simulink model "shabih_model"  (R2021a)
settings: Solver=VariableStepAuto  StartTime=0.0  StopTime=20  MaxStep=0.1  RelTol=1e-3
libraries: cstblocks x3, pid_lib x1
settings Model: Creator=saeed  LastModifiedBy=saeed

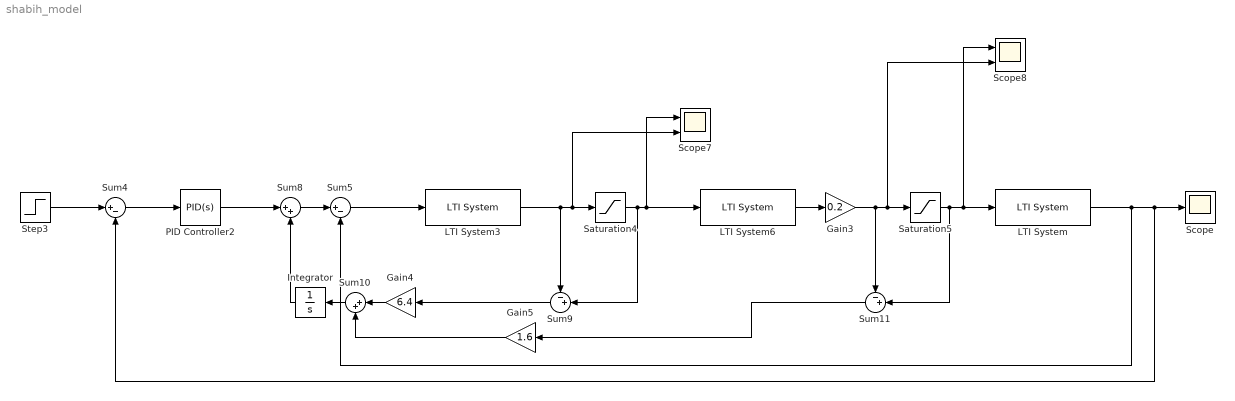
== system shabih_model ==
  Gain3 : Gain  Gain=0.2
  Gain4 : Gain  Gain=6.4
  Gain5 : Gain  Gain=1.6
  Integrator : Integrator
  LTI System : cstblocks/LTI System  sys=G_plant  IC=[]
  LTI System3 : cstblocks/LTI System  sys=C  IC=[]
  LTI System6 : cstblocks/LTI System  sys=G_motor  IC=[]
  PID Controller2 : pid_lib/PID Controller  Controller=PID  Form=Parallel  TimeDomain=Continuous-time  UseExternalTs=off  SampleTime=-1  IntegratorMethod=Forward Euler  FilterMethod=Forward Euler  ControllerParametersSource=internal  P=0.191923492855687  I=0.488933359561099  D=0  UseFilter=on  N=100  TunerSelectOption=Transfer Function Based (PID Tuner App)  InitialConditionSource=internal  InitialConditionForIntegrator=0  InitialConditionForFilter=0  DifferentiatorICPrevScaledInput=0  ExternalReset=none  TrackingMode=off  Kt=1  LimitOutput=on  SatLimitsSource=internal  UpperSaturationLimit=inf  LowerSaturationLimit=-inf  LinearizeAsGain=off  AntiWindupMode=none  Kb=1  POutMin=[]  POutMax=[]  IOutMin=[]  IOutMax=[]  DOutMin=[]  DOutMax=[]  NOutMin=[]  NOutMax=[]  SumOutMin=[]  SumOutMax=[]  SaturationOutMin=[]  SaturationOutMax=[]  PParamMin=[]  PParamMax=[]  IParamMin=[]  IParamMax=[]  DParamMin=[]  DParamMax=[]  NParamMin=[]  NParamMax=[]  KbParamMin=[]  KbParamMax=[]  KtParamMin=[]  KtParamMax=[]  KbOutMin=[]  KbOutMax=[]  KtOutMin=[]  KtOutMax=[]  IntegratorOutMin=[]  IntegratorOutMax=[]  FilterOutMin=[]  FilterOutMax=[]  SumI1OutMin=[]  SumI1OutMax=[]  SumI2OutMin=[]  SumI2OutMax=[]  SumI3OutMin=[]  SumI3OutMax=[]  SumI4OutMin=[]  SumI4OutMax=[]  SumDOutMin=[]  SumDOutMax=[]  DifferentiatorOutMin=[]  DifferentiatorOutMax=[]  FilterDiffOutCoefMin=[]  FilterDiffOutCoefMax=[]  ReciprocalOutMin=[]  ReciprocalOutMax=[]  SumDenOutMin=[]  SumDenOutMax=[]  SumNumOutMin=[]  SumNumOutMax=[]  DivideOutMin=[]  DivideOutMax=[]  UdiffTsProdOutMin=[]  UdiffTsProdOutMax=[]  NTsProdOutMin=[]  NTsProdOutMax=[]  UintegralTsProdOutMin=[]  UintegralTsProdOutMax=[]  UngainTsProdOutMin=[]  UngainTsProdOutMax=[]  IntegratorContinuousStateAttributes=''  IntegratorStateMustResolveToSignalObject=off  IntegratorRTWStateStorageClass=Auto  FilterContinuousStateAttributes=''  FilterStateMustResolveToSignalObject=off  FilterRTWStateStorageClass=Auto  ParallelPVariant=InternalParameters  IdealPVariant=Disabled  IVariant=InternalParameters  DVariant=InternalParameters  IntegratorVariant=Continuous  SatVariant=Enabled  AWVariant=Passthrough  PCopyVariant=Disabled  TRVariant=Disabled  FdbkBlocksVariant=Forward  IdealPFdbkVariant=Disabled  SatFdbkVariant=Disabled  DerivativeFilterVariant=ContFilter  NVariant=InternalParameters  NCopyVariant=Disabled  FilterICVariant=InternalICsFilter  IntegratorICVariant=InternalICs  ExternalResetVariant=Disabled  TRSumVariant=Passthrough  SumFdbkVariant=Disabled  SumVariant=Sum_PID  TsampFilterVariant=InternalTs  TsampNgainVariant=Passthrough  TsampIntegralVariant=Passthrough  ExternalSaturationOutDataTypeStr=Inherit: Same as second input
  Saturation4 : Saturate  UpperLimit=30  LowerLimit=-30
  Saturation5 : Saturate  UpperLimit=pi*0.47  LowerLimit=-pi*0.47
  Scope : Scope
  Scope7 : Scope  NumInputPorts=2
  Scope8 : Scope  NumInputPorts=2
  Step3 : Step  Time=0  After=1.5  SampleTime=0
  Sum10 : Sum  Inputs=|++
  Sum11 : Sum  Inputs=-+|
  Sum4 : Sum  Inputs=|+-
  Sum5 : Sum  Inputs=|+-
  Sum8 : Sum  Inputs=|++
  Sum9 : Sum  Inputs=-+|
  wires:
  Sum9/1 -> Gain4/1
  LTI System3/1 -> Scope7/2, Saturation4/1, Sum9/1
  LTI System/1 -> Sum5/2, Scope/1, Sum4/2
  Sum4/1 -> PID Controller2/1
  Gain3/1 -> Sum11/1, Scope8/2, Saturation5/1
  Step3/1 -> Sum4/1
  Sum5/1 -> LTI System3/1
  Saturation4/1 -> Sum9/2, Scope7/1, LTI System6/1
  LTI System6/1 -> Gain3/1
  Gain5/1 -> Sum10/2
  Sum10/1 -> Integrator/1
  Sum11/1 -> Gain5/1
  Integrator/1 -> Sum8/2
  Gain4/1 -> Sum10/1
  Sum8/1 -> Sum5/1
  Saturation5/1 -> Sum11/2, LTI System/1, Scope8/1
  PID Controller2/1 -> Sum8/1
